simulink model "IEEE30_case"  (R2024b)
settings: Solver=FixedStepAuto  StartTime=0  StopTime=5  FixedStep=1e-7  RelTol=1e-3
values from neighbouring files (symbols this model uses):
  GFL_DFIG_7_C_bus = 0.08    [IEEE30_case_parameters.m]
  GFL_DFIG_7_D_mutual = 2.500000e+3    (= 2500)    [IEEE30_case_parameters.m]
  GFL_DFIG_7_f0 = 60    [IEEE30_case_parameters.m]
  GFL_DFIG_7_gPLLi = 3200    [IEEE30_case_parameters.m]
  GFL_DFIG_7_gPLLp = 650    [IEEE30_case_parameters.m]
  GFL_DFIG_7_H_WT = 0.4    [IEEE30_case_parameters.m]
  GFL_DFIG_7_Hg = 0.8    [IEEE30_case_parameters.m]
  GFL_DFIG_7_Igq_ref = 0    [IEEE30_case_parameters.m]
  GFL_DFIG_7_Ird_ref = 704.45696    [IEEE30_case_parameters.m]
  GFL_DFIG_7_KI_V = -300000    [IEEE30_case_parameters.m]
  GFL_DFIG_7_KP_V = -1000    [IEEE30_case_parameters.m]
  GFL_DFIG_7_Ksh = 1.254300e+4    (= 12543)    [IEEE30_case_parameters.m]
  GFL_DFIG_7_Lg = 0.000483    [IEEE30_case_parameters.m]
  GFL_DFIG_7_Lm_pu = 4    [IEEE30_case_parameters.m]
  GFL_DFIG_7_N = 100    [IEEE30_case_parameters.m]
  GFL_DFIG_7_p = 2    [IEEE30_case_parameters.m]
  GFL_DFIG_7_Pitch = 0    [IEEE30_case_parameters.m]
  GFL_DFIG_7_R = 44    [IEEE30_case_parameters.m]
  GFL_DFIG_7_Rg = 2.000000e-5    (= 2e-05)    [IEEE30_case_parameters.m]
  GFL_DFIG_7_rho = 1.225    [IEEE30_case_parameters.m]
  GFL_DFIG_7_rPLLi = 4500    [IEEE30_case_parameters.m]
  GFL_DFIG_7_rPLLp = 620    [IEEE30_case_parameters.m]
  GFL_DFIG_7_Rs_pu = 0.011    [IEEE30_case_parameters.m]
  GFL_DFIG_7_Sbase = 2.000000e+6    (= 2000000)    [IEEE30_case_parameters.m]
  GFL_DFIG_7_ugq_ref = 0    [IEEE30_case_parameters.m]
  GFL_DFIG_7_usd_ref = 0    [IEEE30_case_parameters.m]
  GFL_DFIG_7_Vbase = 690    [IEEE30_case_parameters.m]
  GFL_DFIG_7_Vdc_ref = 1200    [IEEE30_case_parameters.m]
  GFL_DFIG_7_wind = 12    [IEEE30_case_parameters.m]
  GFL_DFIG_7_wm_ref = 518.184209    [IEEE30_case_parameters.m]
  SG_D_13_D = 0.01056    [IEEE30_case_parameters.m]
  SG_D_13_EnableSaturation = 0    [IEEE30_case_parameters.m]
  SG_D_13_f0 = 60    [IEEE30_case_parameters.m]
  SG_D_13_H = 7.5    [IEEE30_case_parameters.m]
  SG_D_13_K_A = 20    [IEEE30_case_parameters.m]
  SG_D_13_K_E = 1.000000e+1    (= 10)    [IEEE30_case_parameters.m]
  SG_D_13_K_F = 2.363    [IEEE30_case_parameters.m]
  SG_D_13_K_s = 0.5    [IEEE30_case_parameters.m]
  SG_D_13_R_a = 0.001088    [IEEE30_case_parameters.m]
  SG_D_13_S_A = 1    [IEEE30_case_parameters.m]
  SG_D_13_S_B = 0.103    [IEEE30_case_parameters.m]
  SG_D_13_S_N = 10.659857    [IEEE30_case_parameters.m]
  SG_D_13_SpeedPara = 200    [IEEE30_case_parameters.m]
  SG_D_13_T_0 = 0.370163    [IEEE30_case_parameters.m]
  SG_D_13_T_1 = 0.3    [IEEE30_case_parameters.m]
  SG_D_13_T_2 = 0.05    [IEEE30_case_parameters.m]
  SG_D_13_T_3 = 0.02    [IEEE30_case_parameters.m]
  SG_D_13_T_4 = 0.005    [IEEE30_case_parameters.m]
  SG_D_13_T_A = 0.02    [IEEE30_case_parameters.m]
  SG_D_13_T_dd = 8.000000e+0    (= 8)    [IEEE30_case_parameters.m]
  SG_D_13_T_ddd = 0.04    [IEEE30_case_parameters.m]
  SG_D_13_T_E = 0.314    [IEEE30_case_parameters.m]
  SG_D_13_T_F = 0.35    [IEEE30_case_parameters.m]
  SG_D_13_T_qd = 0.8    [IEEE30_case_parameters.m]
  SG_D_13_T_qdd = 0.02    [IEEE30_case_parameters.m]
  SG_D_13_T_speed = 0.1    [IEEE30_case_parameters.m]
  SG_D_13_T_w = 0.5    [IEEE30_case_parameters.m]
  SG_D_13_V_ref = 1.696619    [IEEE30_case_parameters.m]
  SG_D_13_w_ref = 376.991118    [IEEE30_case_parameters.m]
  SG_D_13_x_d = 1.9    [IEEE30_case_parameters.m]
  SG_D_13_x_dd = 0.302    [IEEE30_case_parameters.m]
  SG_D_13_x_ddd = 0.204    [IEEE30_case_parameters.m]
  SG_D_13_x_l = 0.05    [IEEE30_case_parameters.m]
  SG_D_13_x_q = 1.3    [IEEE30_case_parameters.m]
  SG_D_13_x_qd = 0.5    [IEEE30_case_parameters.m]
  SG_D_13_x_qdd = 0.3    [IEEE30_case_parameters.m]
  SG_D_1_D = 0.01056    [IEEE30_case_parameters.m]
  SG_D_1_EnableSaturation = 0    [IEEE30_case_parameters.m]
  SG_D_1_f0 = 60    [IEEE30_case_parameters.m]
  SG_D_1_H = 7.5    [IEEE30_case_parameters.m]
  SG_D_1_K_A = 20    [IEEE30_case_parameters.m]
  SG_D_1_K_E = 1.000000e+1    (= 10)    [IEEE30_case_parameters.m]
  SG_D_1_K_F = 2.363    [IEEE30_case_parameters.m]
  SG_D_1_K_s = 0.5    [IEEE30_case_parameters.m]
  SG_D_1_R_a = 0.001088    [IEEE30_case_parameters.m]
  SG_D_1_S_A = 1    [IEEE30_case_parameters.m]
  SG_D_1_S_B = 0.103    [IEEE30_case_parameters.m]
  SG_D_1_S_N = 10.659857    [IEEE30_case_parameters.m]
  SG_D_1_SpeedPara = 200    [IEEE30_case_parameters.m]
  SG_D_1_T_0 = 0.259812    [IEEE30_case_parameters.m]
  SG_D_1_T_1 = 0.3    [IEEE30_case_parameters.m]
  SG_D_1_T_2 = 0.05    [IEEE30_case_parameters.m]
  SG_D_1_T_3 = 0.02    [IEEE30_case_parameters.m]
  SG_D_1_T_4 = 0.005    [IEEE30_case_parameters.m]
  SG_D_1_T_A = 0.02    [IEEE30_case_parameters.m]
  SG_D_1_T_dd = 8.000000e+0    (= 8)    [IEEE30_case_parameters.m]
  SG_D_1_T_ddd = 0.04    [IEEE30_case_parameters.m]
  SG_D_1_T_E = 0.314    [IEEE30_case_parameters.m]
  SG_D_1_T_F = 0.35    [IEEE30_case_parameters.m]
  SG_D_1_T_qd = 0.8    [IEEE30_case_parameters.m]
  SG_D_1_T_qdd = 0.02    [IEEE30_case_parameters.m]
  SG_D_1_T_speed = 0.1    [IEEE30_case_parameters.m]
  SG_D_1_T_w = 0.5    [IEEE30_case_parameters.m]
  SG_D_1_V_ref = 1.544107    [IEEE30_case_parameters.m]
  SG_D_1_w_ref = 376.991118    [IEEE30_case_parameters.m]
  SG_D_1_x_d = 1.9    [IEEE30_case_parameters.m]
  SG_D_1_x_dd = 0.302    [IEEE30_case_parameters.m]
  SG_D_1_x_ddd = 0.204    [IEEE30_case_parameters.m]
  SG_D_1_x_l = 0.05    [IEEE30_case_parameters.m]
  SG_D_1_x_q = 1.3    [IEEE30_case_parameters.m]
  SG_D_1_x_qd = 0.5    [IEEE30_case_parameters.m]
  SG_D_1_x_qdd = 0.3    [IEEE30_case_parameters.m]
  SG_D_22_D = 0.01056    [IEEE30_case_parameters.m]
  SG_D_22_EnableSaturation = 0    [IEEE30_case_parameters.m]
  SG_D_22_f0 = 60    [IEEE30_case_parameters.m]
  SG_D_22_H = 7.5    [IEEE30_case_parameters.m]
  SG_D_22_K_A = 20    [IEEE30_case_parameters.m]
  SG_D_22_K_E = 1.000000e+1    (= 10)    [IEEE30_case_parameters.m]
  SG_D_22_K_F = 2.363    [IEEE30_case_parameters.m]
  SG_D_22_K_s = 0.5    [IEEE30_case_parameters.m]
  SG_D_22_R_a = 0.001088    [IEEE30_case_parameters.m]
  SG_D_22_S_A = 1    [IEEE30_case_parameters.m]
  SG_D_22_S_B = 0.103    [IEEE30_case_parameters.m]
  SG_D_22_S_N = 10.659857    [IEEE30_case_parameters.m]
  SG_D_22_SpeedPara = 200    [IEEE30_case_parameters.m]
  SG_D_22_T_0 = 0.216121    [IEEE30_case_parameters.m]
  SG_D_22_T_1 = 0.3    [IEEE30_case_parameters.m]
  SG_D_22_T_2 = 0.05    [IEEE30_case_parameters.m]
  SG_D_22_T_3 = 0.02    [IEEE30_case_parameters.m]
  SG_D_22_T_4 = 0.005    [IEEE30_case_parameters.m]
  ... (+126 more)
(part 15 of 27)

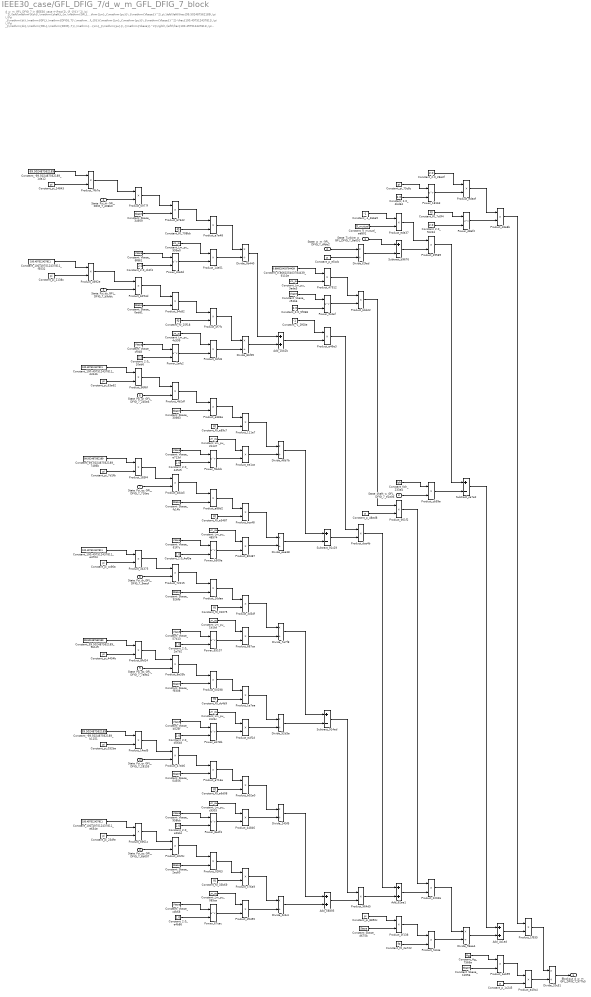
== system IEEE30_case/GFL_DFIG_7/d_w_m_GFL_DFIG_7_block ==
  note: d_w_m_GFL_DFIG_7 in IEEE30_case
      | $-\frac{2\,{f_{0}}^2\,\pi ^2\,\left(\mathrm{Ksh}\,\mathrm{shaft}_{w,\mathrm{GFL},\mathrm{DFIG},7}+D_{\mathrm{mutual}}\,\left(\mathrm{Turbine}_{w,\mathrm{GFL},\mathrm{DFIG},7}-\frac{w_{m,\mathrm{GFL},\mathrm{DFIG},7}}{p}\right)-\frac{0.866025403784439\,\mathrm{Lm}_{\mathrm{pu}}\,{\mathrm{Vbase}}^2\,p\,\left(\left(\frac{99.502487562189\,\pi \,\Psi _{\mathrm{dr},\mathrm{GFL},\mathrm{DFIG},7}\,\mathrm{Sbase}\,f_{0}}{\mathrm{Lm}_{\mathrm{pu}}\,{\mathrm{Vbase}}^2}-\frac{100.497512437811\,\pi \,\Psi _{\mathrm{ds},\mathrm{GFL},\mathrm{DFIG},7}\,\mathrm{Sbase}\,f_{0}}{\mathrm{Lm}_{\mathrm{pu}}\,{\mathrm{Vbase}}^2}\right)\,\left(\frac{100.497512437811\,\pi \,\Psi _{\mathrm{qr},\mathrm{GFL},\mathrm{DFIG},7}\,\mathrm{Sbase}\,f_{0}}{\mathrm{Lm}_{\mathrm{pu}}\,{\mathrm{Vbase}}^2}-\frac{99.502487562189\,\pi \,\Psi _{\mathrm{qs},\mathrm{GFL},\mathrm{DFIG},7}\,\mathrm{Sbase}\,f_{0}}{\mathrm{Lm}_{\mathrm{pu}}\,{\mathrm{Vbase}}^2}\right)-\left(\frac{100.497512437811\,\pi \,\Psi _{\mathrm{dr},\mathrm{GFL},\mathrm{DFIG},7}\,\mathrm{Sbase}\,f_{0}}{\mathrm{Lm}_{\mathrm{pu}}\,{\mathrm{Vbase}}^2}-\frac{99.502487562189\,\pi \,\Psi _{\mathrm{ds},\mathrm{GFL},\mathrm{DFIG},7}\,\mathrm{Sbase}\,f_{0}}{\mathrm{Lm}_{\mathrm{pu}}\,{\mathrm{Vbase}}^2}\right)\,\left(\frac{99.502487562189\,\pi \,\Psi _{\mathrm{qr},\mathrm{GFL},\mathrm{DFIG},7}\,\mathrm{Sbase}\,f_{0}}{\mathrm{Lm}_{\mathrm{pu}}\,{\mathrm{Vbase}}^2}-\frac{100.497512437811\,\pi \,\Psi _{\mathrm{qs},\mathrm{GFL},\mathrm{DFIG},7}\,\mathrm{Sbase}\,f_{0}}{\mathrm{Lm}_{\mathrm{pu}}\,{\mathrm{Vbase}}^2}\right)\right)}{\mathrm{Sbase}\,f_{0}\,\pi }\right)}{\mathrm{Hg}\,\mathrm{Sbase}\,p}$
      | Automatically generated on 2025-11-01 18:32:24 .
  State_Turbine_w_GFL_DFIG_7_8e651 : Inport
  State_w_m_GFL_DFIG_7_dfde2 : Inport  Port=2
  State_shaft_w_GFL_DFIG_7_e1a06 : Inport  Port=3
  State_Psi_dr_GFL_DFIG_7_d08b0 : Inport  Port=4
  State_Psi_ds_GFL_DFIG_7_b9ddc : Inport  Port=5
  State_Psi_qr_GFL_DFIG_7_240a6 : Inport  Port=6
  State_Psi_qs_GFL_DFIG_7_716ac : Inport  Port=7
  State_Psi_dr_GFL_DFIG_7_9aecf : Inport  Port=8
  State_Psi_ds_GFL_DFIG_7_7aea2 : Inport  Port=9
  State_Psi_qr_GFL_DFIG_7_28155 : Inport  Port=10
  State_Psi_qs_GFL_DFIG_7_6b007 : Inport  Port=11
  Add_1bb2b : Sum
  Add_4c1ed : Sum
  Add_58d95 : Sum
  Add_62ae1 : Sum
  Constant_-1_2f60e : Constant  Value=-1
  Constant_-1_466a5 : Constant  Value=-1
  Constant_-99.502487562189_1da12 : Constant  Value=-99.502487562189
  Constant_-99.502487562189_b1151 : Constant  Value=-99.502487562189
  Constant_0.866025403784439_9110e : Constant  Value=0.866025403784439
  Constant_100.497512437811_dd14b : Constant  Value=100.497512437811
  Constant_100.497512437811_e4704 : Constant  Value=100.497512437811
  Constant_100.497512437811_e654e : Constant  Value=100.497512437811
  Constant_100.497512437811_f5532 : Constant  Value=100.497512437811
  Constant_2.0_10ab6 : Constant  Value=2.0
  Constant_2.0_28e3f : Constant  Value=2.0
  Constant_2.0_2a7b2 : Constant  Value=2.0
  Constant_2.0_445c5 : Constant  Value=2.0
  Constant_2.0_4bd64 : Constant  Value=2.0
  Constant_2.0_4ef5a : Constant  Value=2.0
  Constant_2.0_5f068 : Constant  Value=2.0
  Constant_2.0_9c243 : Constant  Value=2.0
  Constant_2.0_cb1f4 : Constant  Value=2.0
  Constant_2.0_d56bd : Constant  Value=2.0
  Constant_2.0_e26bc : Constant  Value=2.0
  Constant_2.0_e4b86 : Constant  Value=2.0
  Constant_99.502487562189_7486b : Constant  Value=99.502487562189
  Constant_99.502487562189_9b1c9 : Constant  Value=99.502487562189
  Constant_D_mutual_aed01 : Constant  Value=D_mutual
  Constant_Hg_7566a : Constant  Value=Hg
  Constant_Ksh_233a4 : Constant  Value=Ksh
  Constant_Lm_pu_085ca : Constant  Value=Lm_pu
  Constant_Lm_pu_1b1cd : Constant  Value=Lm_pu
  Constant_Lm_pu_2b137 : Constant  Value=Lm_pu
  Constant_Lm_pu_2c24c : Constant  Value=Lm_pu
  Constant_Lm_pu_3ade3 : Constant  Value=Lm_pu
  Constant_Lm_pu_48574 : Constant  Value=Lm_pu
  Constant_Lm_pu_4c599 : Constant  Value=Lm_pu
  Constant_Lm_pu_999a0 : Constant  Value=Lm_pu
  Constant_Lm_pu_c9303 : Constant  Value=Lm_pu
  Constant_Sbase_04556 : Constant  Value=Sbase
  Constant_Sbase_0add1 : Constant  Value=Sbase
  Constant_Sbase_1b556 : Constant  Value=Sbase
  Constant_Sbase_2ec60 : Constant  Value=Sbase
  Constant_Sbase_30983 : Constant  Value=Sbase
  Constant_Sbase_34959 : Constant  Value=Sbase
  Constant_Sbase_926fb : Constant  Value=Sbase
  Constant_Sbase_d675b : Constant  Value=Sbase
  Constant_Sbase_f9308 : Constant  Value=Sbase
  Constant_Sbase_fc14b : Constant  Value=Sbase
  Constant_Vbase_57b13 : Constant  Value=Vbase
  Constant_Vbase_61f7c : Constant  Value=Vbase
  Constant_Vbase_6f861 : Constant  Value=Vbase
  Constant_Vbase_958bb : Constant  Value=Vbase
  Constant_Vbase_b526f : Constant  Value=Vbase
  Constant_Vbase_c53b6 : Constant  Value=Vbase
  Constant_Vbase_cdb68 : Constant  Value=Vbase
  Constant_Vbase_cf948 : Constant  Value=Vbase
  Constant_Vbase_e713d : Constant  Value=Vbase
  Constant_f0_01075 : Constant  Value=f0
  Constant_f0_25f18 : Constant  Value=f0
  Constant_f0_2e722 : Constant  Value=f0
  Constant_f0_33b69 : Constant  Value=f0
  Constant_f0_708bb : Constant  Value=f0
  Constant_f0_7c0f4 : Constant  Value=f0
  Constant_f0_a3487 : Constant  Value=f0
  Constant_f0_a6d08 : Constant  Value=f0
  Constant_f0_dc4b9 : Constant  Value=f0
  Constant_f0_e89c7 : Constant  Value=f0
  Constant_p_1c245 : Constant  Value=p
  Constant_p_48ad8 : Constant  Value=p
  Constant_p_e5cdc : Constant  Value=p
  Constant_pi_032ba : Constant  Value=pi
  Constant_pi_2138c : Constant  Value=pi
  Constant_pi_23dfe : Constant  Value=pi
  Constant_pi_24843 : Constant  Value=pi
  Constant_pi_4454b : Constant  Value=pi
  Constant_pi_63a62 : Constant  Value=pi
  Constant_pi_75c8c : Constant  Value=pi
  Constant_pi_7d1fb : Constant  Value=pi
  Constant_pi_8850c : Constant  Value=pi
  Constant_pi_cc96a : Constant  Value=pi
  Divide_0b440 : Product  Inputs=*/
  Divide_0c4cc : Product  Inputs=*/
  Divide_20c51 : Product  Inputs=*/
  Divide_245f5 : Product  Inputs=*/
  Divide_46b7b : Product  Inputs=*/
  Divide_52d3a : Product  Inputs=*/
  Divide_7e7f8 : Product  Inputs=*/
  Divide_8bf05 : Product  Inputs=*/
  Divide_96aa4 : Product  Inputs=*/
  Divide_eaa38 : Product  Inputs=*/
  Divide_f2fed : Product  Inputs=*/
  Power_18163 : Math  Operator=pow
  Power_2afc2 : Math  Operator=pow
  Power_3ca0d : Math  Operator=pow
  Power_65107 : Math  Operator=pow
  Power_67cac : Math  Operator=pow
  Power_8adf3 : Math  Operator=pow
  Power_9bdcb : Math  Operator=pow
  Power_9c4ef : Math  Operator=pow
  Power_b500e : Math  Operator=pow
  Power_d8ef2 : Math  Operator=pow
  Power_eb78b : Math  Operator=pow
  Product_00298 : Product
  Product_02f63 : Product
  Product_0977f : Product
  Product_0cfc8 : Product
  Product_111e7 : Product
  Product_14ad5 : Product
  Product_14e51 : Product
  Product_16daa : Product
  Product_183f4 : Product
  Product_1e7aa : Product
  Product_1eb99 : Product
  Product_1f935 : Product
  Product_{22046,34375,44846,47912,49589,67642,72215,80487} (8 alike) : Product
  Product_3d3df : Product
  Product_3f138 : Product
  Product_47ab6 : Product
  Product_484c5 : Product
  Product_4992e : Product
  Product_4b2df : Product
  Product_4f7fc : Product
  Product_6294d : Product
  Product_7fb7e : Product
  Product_887ca : Product
  Product_8a33b : Product
  Product_8fd24 : Product
  Product_901f2 : Product
  Product_94c82 : Product
  Product_964d5 : Product
  Product_96f6f : Product
  Product_a49c4 : Product
  Product_a4f1d : Product
  Product_a716a : Product
  Product_a88d2 : Product
  Product_b02a0 : Product
  Product_b961c : Product
  Product_bbb22 : Product
  Product_bcc48 : Product
  Product_c76a9 : Product
  Product_cb99a : Product
  Product_d2c5c : Product
  Product_d3a8b : Product
  Product_d5455 : Product
  Product_dce4b : Product
  Product_e383e : Product
  Product_e46e3 : Product
  Product_e7a48 : Product
  Product_eda37 : Product
  Product_edaaf : Product
  Product_ee1ca : Product
  Product_f4c4e : Product
  Subtract_914ed : Sum  Inputs=+-
  Subtract_91c29 : Sum  Inputs=+-
  Subtract_b9676 : Sum  Inputs=+-
  Subtract_ca7e2 : Sum  Inputs=+-
  Blockout_d_w_m_GFL_DFIG_7_977b5 : Outport
  wires:
  Product_1eb99/1 -> Product_a49c4/1
  Add_4c1ed/1 -> Product_1f935/2
  Divide_20c51/1 -> Blockout_d_w_m_GFL_DFIG_7_977b5/1
  Product_16daa/1 -> Product_3d3df/1
  Constant_2.0_4ef5a/1 -> Power_b500e/2
  Constant_-99.502487562189_b1151/1 -> Product_14ad5/1
  Add_62ae1/1 -> Product_22046/2
  Product_a49c4/1 -> Divide_20c51/2
  Constant_Vbase_b526f/1 -> Power_eb78b/1
  Constant_-1_2f60e/1 -> Product_e46e3/1
  Product_44846/1 -> Divide_245f5/2
  Product_22046/1 -> Divide_96aa4/1
  Product_1f935/1 -> Divide_20c51/1
  Constant_p_1c245/1 -> Product_a49c4/2
  Constant_99.502487562189_9b1c9/1 -> Product_8fd24/1
  Add_58d95/1 -> Product_964d5/2
  Product_964d5/1 -> Add_62ae1/2
  Product_f4c4e/1 -> Divide_96aa4/2
  Product_d5455/1 -> Divide_0c4cc/2
  Subtract_91c29/1 -> Product_dce4b/2
  Constant_2.0_4bd64/1 -> Power_18163/2
  Constant_Sbase_1b556/1 -> Product_1eb99/2
  Divide_eaa38/1 -> Subtract_91c29/2
  Constant_Hg_7566a/1 -> Product_1eb99/1
  Constant_Sbase_2ec60/1 -> Product_02f63/2
  Constant_Vbase_958bb/1 -> Power_8adf3/1
  Divide_0c4cc/1 -> Add_58d95/2
  Constant_2.0_28e3f/1 -> Product_edaaf/1
  Product_a4f1d/1 -> Divide_52d3a/2
  Constant_Lm_pu_48574/1 -> Product_80487/1
  Constant_Sbase_30983/1 -> Product_e383e/2
  Product_b961c/1 -> Product_d2c5c/1
  State_shaft_w_GFL_DFIG_7_e1a06/1 -> Product_cb99a/2
  Divide_96aa4/1 -> Add_4c1ed/2
  Constant_Lm_pu_2c24c/1 -> Product_a4f1d/1
  Constant_Sbase_926fb/1 -> Product_16daa/2
  Product_d2c5c/1 -> Product_02f63/1
  Product_c76a9/1 -> Divide_0c4cc/1
  Power_9c4ef/1 -> Product_bbb22/2
  Constant_pi_8850c/1 -> Product_3f138/1
  Constant_f0_2e722/1 -> Product_f4c4e/2
  Constant_f0_e89c7/1 -> Product_111e7/2
  Product_3f138/1 -> Product_f4c4e/1
  Product_4b2df/1 -> Product_e383e/1
  Constant_2.0_e26bc/1 -> Power_8adf3/2
  State_Psi_dr_GFL_DFIG_7_d08b0/1 -> Product_0977f/2
  Constant_Sbase_d675b/1 -> Product_3f138/2
  Product_8a33b/1 -> Product_00298/1
  Constant_pi_032ba/1 -> Product_14ad5/2
  Constant_Vbase_cdb68/1 -> Power_67cac/1
  Divide_245f5/1 -> Add_58d95/1
  Constant_Lm_pu_c9303/1 -> Product_44846/1
  Product_3d3df/1 -> Divide_7e7f8/1
  Power_67cac/1 -> Product_d5455/2
  State_Psi_ds_GFL_DFIG_7_7aea2/1 -> Product_8a33b/2
  Product_96f6f/1 -> Product_4b2df/1
  Constant_2.0_e4b86/1 -> Power_67cac/2
  Divide_8bf05/1 -> Add_1bb2b/2
  Constant_Lm_pu_085ca/1 -> Product_d5455/1
  Constant_pi_2138c/1 -> Product_4992e/2
  Constant_f0_33b69/1 -> Product_c76a9/2
  Product_02f63/1 -> Product_c76a9/1
  Power_8adf3/1 -> Product_44846/2
  State_Psi_qs_GFL_DFIG_7_6b007/1 -> Product_d2c5c/2
  Constant_100.497512437811_e654e/1 -> Product_b961c/1
  Constant_Sbase_f9308/1 -> Product_00298/2
  Constant_pi_23dfe/1 -> Product_b961c/2
  Product_8fd24/1 -> Product_8a33b/1
  State_Psi_qr_GFL_DFIG_7_28155/1 -> Product_47ab6/2
  State_Psi_qs_GFL_DFIG_7_716ac/1 -> Product_484c5/2
  State_Turbine_w_GFL_DFIG_7_8e651/1 -> Subtract_b9676/1
  Constant_Sbase_fc14b/1 -> Product_a88d2/2
  Product_b02a0/1 -> Divide_245f5/1
  Power_eb78b/1 -> Product_a4f1d/2
  Subtract_914ed/1 -> Product_964d5/1
  Constant_f0_a6d08/1 -> Product_b02a0/2
  Product_a716a/1 -> Product_b02a0/1
  Constant_2.0_5f068/1 -> Power_9c4ef/2
  Constant_Sbase_04556/1 -> Product_a716a/2
  Constant_f0_dc4b9/1 -> Product_1e7aa/2
  Product_47ab6/1 -> Product_a716a/1
  Product_eda37/1 -> Product_49589/1
  Product_80487/1 -> Divide_eaa38/2
  Product_14ad5/1 -> Product_47ab6/1
  Product_00298/1 -> Product_1e7aa/1
  Divide_52d3a/1 -> Subtract_914ed/2
  Constant_2.0_d56bd/1 -> Power_eb78b/2
  Product_1e7aa/1 -> Divide_52d3a/1
  Constant_pi_4454b/1 -> Product_8fd24/2
  Divide_7e7f8/1 -> Subtract_914ed/1
  Product_887ca/1 -> Divide_7e7f8/2
  Power_65107/1 -> Product_887ca/2
  Constant_pi_75c8c/1 -> Power_18163/1
  Constant_2.0_2a7b2/1 -> Power_65107/2
  Constant_Vbase_57b13/1 -> Power_65107/1
  Constant_Lm_pu_1b1cd/1 -> Product_887ca/1
  Constant_f0_01075/1 -> Product_3d3df/2
  Product_72215/1 -> Product_16daa/1
  State_Psi_dr_GFL_DFIG_7_9aecf/1 -> Product_72215/2
  Product_34375/1 -> Product_72215/1
  Constant_pi_cc96a/1 -> Product_34375/2
  Constant_100.497512437811_e4704/1 -> Product_34375/1
  Product_d3a8b/1 -> Product_1f935/1
  Product_dce4b/1 -> Add_62ae1/1
  Power_b500e/1 -> Product_80487/2
  Constant_Vbase_61f7c/1 -> Power_b500e/1
  Product_bcc48/1 -> Divide_eaa38/1
  Constant_f0_a3487/1 -> Product_bcc48/2
  Product_a88d2/1 -> Product_bcc48/1
  Subtract_ca7e2/1 -> Add_4c1ed/1
  Product_484c5/1 -> Product_a88d2/1
  Product_183f4/1 -> Product_484c5/1
  Constant_2.0_9c243/1 -> Power_d8ef2/2
  Constant_pi_7d1fb/1 -> Product_183f4/2
  Constant_99.502487562189_7486b/1 -> Product_183f4/1
  Divide_46b7b/1 -> Subtract_91c29/1
  Divide_f2fed/1 -> Subtract_b9676/2
  Product_ee1ca/1 -> Divide_46b7b/2
  Power_9bdcb/1 -> Product_ee1ca/2
  Constant_2.0_445c5/1 -> Power_9bdcb/2
  Constant_Vbase_e713d/1 -> Power_9bdcb/1
  State_w_m_GFL_DFIG_7_dfde2/1 -> Divide_f2fed/1
  Constant_Lm_pu_2b137/1 -> Product_ee1ca/1
  Product_111e7/1 -> Divide_46b7b/1
  Product_e383e/1 -> Product_111e7/1
  State_Psi_qr_GFL_DFIG_7_240a6/1 -> Product_4b2df/2
  Constant_pi_63a62/1 -> Product_96f6f/2
  Constant_100.497512437811_dd14b/1 -> Product_96f6f/1
  Product_e46e3/1 -> Product_dce4b/1
  Add_1bb2b/1 -> Product_e46e3/2
  Product_0cfc8/1 -> Divide_8bf05/2
  Power_2afc2/1 -> Product_0cfc8/2
  Constant_2.0_10ab6/1 -> Power_2afc2/2
  Constant_Vbase_cf948/1 -> Power_2afc2/1
  Constant_Sbase_34959/1 -> Product_67642/2
  Constant_Lm_pu_4c599/1 -> Product_0cfc8/1
  Product_e7a48/1 -> Divide_0b440/1
  Product_4f7fc/1 -> Divide_8bf05/1
  Constant_f0_25f18/1 -> Product_4f7fc/2
  Product_94c82/1 -> Product_4f7fc/1
  Constant_Sbase_0add1/1 -> Product_94c82/2
  Product_6294d/1 -> Product_94c82/1
  State_Psi_ds_GFL_DFIG_7_b9ddc/1 -> Product_6294d/2
  Product_4992e/1 -> Product_6294d/1
  Constant_100.497512437811_f5532/1 -> Product_4992e/1
  Divide_0b440/1 -> Add_1bb2b/1
  Product_14e51/1 -> Divide_0b440/2
  Power_3ca0d/1 -> Product_14e51/2
  Constant_2.0_cb1f4/1 -> Power_3ca0d/2
  Constant_Vbase_6f861/1 -> Power_3ca0d/1
  Constant_Lm_pu_999a0/1 -> Product_14e51/1
  Constant_f0_708bb/1 -> Product_e7a48/2
  Product_67642/1 -> Product_e7a48/1
  Constant_p_e5cdc/1 -> Divide_f2fed/2
  Product_0977f/1 -> Product_67642/1
  Product_7fb7e/1 -> Product_0977f/1
  Constant_pi_24843/1 -> Product_7fb7e/2
  Constant_-99.502487562189_1da12/1 -> Product_7fb7e/1
  Product_901f2/1 -> Product_22046/1
  Constant_p_48ad8/1 -> Product_901f2/2
  Product_bbb22/1 -> Product_901f2/1
  Constant_Vbase_c53b6/1 -> Power_9c4ef/1
  Product_47912/1 -> Product_bbb22/1
  Constant_Lm_pu_3ade3/1 -> Product_47912/2
  Constant_0.866025403784439_9110e/1 -> Product_47912/1
  Product_cb99a/1 -> Subtract_ca7e2/2
  Constant_Ksh_233a4/1 -> Product_cb99a/1
  Product_49589/1 -> Subtract_ca7e2/1
  Subtract_b9676/1 -> Product_49589/2
  Constant_D_mutual_aed01/1 -> Product_eda37/2
  Constant_-1_466a5/1 -> Product_eda37/1
  Power_d8ef2/1 -> Product_d3a8b/2
  Constant_f0_7c0f4/1 -> Power_d8ef2/1
  Product_edaaf/1 -> Product_d3a8b/1
  Power_18163/1 -> Product_edaaf/2

== system IEEE30_case/GFL_DFIG_7/i_d_GFL_DFIG_7_block ==
  note: i_d_GFL_DFIG_7 in IEEE30_case
      | $-\frac{0.0000345\,\mathrm{Sbase}\,\left(\frac{1.73205080756888\,\mathrm{Vbase}\,\left(\cos\left(\theta _{\mathrm{pllr},\mathrm{GFL},\mathrm{DFIG},7}\right)\,\left(\frac{99.502487562189\,\pi \,\Psi _{\mathrm{dr},\mathrm{GFL},\mathrm{DFIG},7}\,\mathrm{Sbase}\,f_{0}}{\mathrm{Lm}_{\mathrm{pu}}\,{\mathrm{Vbase}}^2}-\frac{100.497512437811\,\pi \,\Psi _{\mathrm{ds},\mathrm{GFL},\mathrm{DFIG},7}\,\mathrm{Sbase}\,f_{0}}{\mathrm{Lm}_{\mathrm{pu}}\,{\mathrm{Vbase}}^2}\right)+\sin\left(\theta _{\mathrm{pllr},\mathrm{GFL},\mathrm{DFIG},7}\right)\,\left(\frac{99.502487562189\,\pi \,\Psi _{\mathrm{qr},\mathrm{GFL},\mathrm{DFIG},7}\,\mathrm{Sbase}\,f_{0}}{\mathrm{Lm}_{\mathrm{pu}}\,{\mathrm{Vbase}}^2}-\frac{100.497512437811\,\pi \,\Psi _{\mathrm{qs},\mathrm{GFL},\mathrm{DFIG},7}\,\mathrm{Sbase}\,f_{0}}{\mathrm{Lm}_{\mathrm{pu}}\,{\mathrm{Vbase}}^2}\right)\right)}{\mathrm{Sbase}}-\frac{1.73205080756888\,\mathrm{Vbase}\,\left(i_{\mathrm{gd},\mathrm{GFL},\mathrm{DFIG},7}\,\cos\left(\theta _{\mathrm{pllg},\mathrm{GFL},\mathrm{DFIG},7}\right)+i_{\mathrm{gq},\mathrm{GFL},\mathrm{DFIG},7}\,\sin\left(\theta _{\mathrm{pllg},\mathrm{GFL},\mathrm{DFIG},7}\right)\right)}{\mathrm{Sbase}}\right)}{\mathrm{Vbase}}$
      | Automatically generated on 2025-11-01 18:34:14 .
  State_i_gd_GFL_DFIG_7_c7c38 : Inport
  State_theta_pllg_GFL_DFIG_7_3c4e6 : Inport  Port=2
  State_i_gq_GFL_DFIG_7_12231 : Inport  Port=3
  State_theta_pllg_GFL_DFIG_7_99cce : Inport  Port=4
  State_Psi_dr_GFL_DFIG_7_47f96 : Inport  Port=5
  State_Psi_ds_GFL_DFIG_7_8722f : Inport  Port=6
  State_theta_pllr_GFL_DFIG_7_79db7 : Inport  Port=7
  State_Psi_qr_GFL_DFIG_7_2c5a7 : Inport  Port=8
  State_Psi_qs_GFL_DFIG_7_a1324 : Inport  Port=9
  State_theta_pllr_GFL_DFIG_7_e04ad : Inport  Port=10
  Add_492a2 : Sum
  Add_49bd1 : Sum
  Add_e7d18 : Sum
  Constant_-1_c11df : Constant  Value=-1
  Constant_-5.0_f5269 : Constant  Value=-5.0
  Constant_-99.502487562189_65d39 : Constant  Value=-99.502487562189
  Constant_-99.502487562189_e1ca6 : Constant  Value=-99.502487562189
  Constant_1.73205080756888_ce066 : Constant  Value=1.73205080756888
  Constant_1.73205080756888_e9173 : Constant  Value=1.73205080756888
  Constant_10.0_49afa : Constant  Value=10.0
  Constant_100.497512437811_8d135 : Constant  Value=100.497512437811
  Constant_100.497512437811_9df18 : Constant  Value=100.497512437811
  Constant_2.0_2fdd8 : Constant  Value=2.0
  Constant_2.0_40610 : Constant  Value=2.0
  Constant_2.0_40c81 : Constant  Value=2.0
  Constant_2.0_c02d0 : Constant  Value=2.0
  Constant_3.45_a6674 : Constant  Value=3.45
  Constant_Lm_pu_2dd3f : Constant  Value=Lm_pu
  Constant_Lm_pu_78702 : Constant  Value=Lm_pu
  Constant_Lm_pu_cb21c : Constant  Value=Lm_pu
  Constant_Lm_pu_edadb : Constant  Value=Lm_pu
  Constant_Sbase_0edc5 : Constant  Value=Sbase
  Constant_Sbase_30f20 : Constant  Value=Sbase
  Constant_Sbase_5a1d3 : Constant  Value=Sbase
  Constant_Sbase_9d97b : Constant  Value=Sbase
  Constant_Sbase_d8b83 : Constant  Value=Sbase
  Constant_Sbase_de693 : Constant  Value=Sbase
  Constant_Sbase_fbf63 : Constant  Value=Sbase
  Constant_Vbase_00e0b : Constant  Value=Vbase
  Constant_Vbase_4dc36 : Constant  Value=Vbase
  Constant_Vbase_65299 : Constant  Value=Vbase
  Constant_Vbase_67351 : Constant  Value=Vbase
  Constant_Vbase_97988 : Constant  Value=Vbase
  Constant_Vbase_f62ff : Constant  Value=Vbase
  Constant_Vbase_fa0fe : Constant  Value=Vbase
  Constant_f0_58a72 : Constant  Value=f0
  Constant_f0_75a91 : Constant  Value=f0
  Constant_f0_844bc : Constant  Value=f0
  Constant_f0_94819 : Constant  Value=f0
  Constant_pi_0046d : Constant  Value=pi
  Constant_pi_07071 : Constant  Value=pi
  Constant_pi_98dd5 : Constant  Value=pi
  Constant_pi_ee553 : Constant  Value=pi
  Divide_1a3a0 : Product  Inputs=*/
  Divide_7078c : Product  Inputs=*/
  Divide_7cc1f : Product  Inputs=*/
  Divide_9a0f6 : Product  Inputs=*/
  Divide_c73cd : Product  Inputs=*/
  Divide_d7e58 : Product  Inputs=*/
  Divide_ed1b1 : Product  Inputs=*/
  MathFunc_cos_b7057 : Trigonometry  Operator=cos
  MathFunc_cos_c2863 : Trigonometry  Operator=cos
  MathFunc_sin_bdbfa : Trigonometry
  MathFunc_sin_fb6a3 : Trigonometry
  Power_4816e : Math  Operator=pow
  Power_82469 : Math  Operator=pow
  Power_8f089 : Math  Operator=pow
  Power_98ba8 : Math  Operator=pow
  Power_9e004 : Math  Operator=pow
  Product_07985 : Product
  Product_0fc16 : Product
  Product_1b707 : Product
  Product_24ce9 : Product
  Product_2c6cc : Product
  Product_31851 : Product
  Product_38eb7 : Product
  Product_3fff3 : Product
  Product_4f502 : Product
  Product_5ad5c : Product
  Product_5c8fa : Product
  Product_653a1 : Product
  Product_6c949 : Product
  Product_71635 : Product
  Product_7859f : Product
  Product_7fea7 : Product
  Product_925c3 : Product
  Product_a23e8 : Product
  Product_a2ec9 : Product
  Product_a485c : Product
  Product_aeb12 : Product
  Product_b0865 : Product
  Product_b1903 : Product
  Product_b70ed : Product
  Product_beed1 : Product
  Product_c30f9 : Product
  Product_db37c : Product
  Product_de865 : Product
  Product_dfd1d : Product
  Product_e0cff : Product
  Product_e5dbc : Product
  Product_fe51d : Product
  Subtract_62b79 : Sum  Inputs=+-
  Subtract_a4cea : Sum  Inputs=+-
  Blockout_i_d_GFL_DFIG_7_2a8ae : Outport
  wires:
  Constant_-99.502487562189_e1ca6/1 -> Product_7859f/1
  State_Psi_dr_GFL_DFIG_7_47f96/1 -> Product_5ad5c/2
  Constant_100.497512437811_9df18/1 -> Product_fe51d/1
  State_Psi_ds_GFL_DFIG_7_8722f/1 -> Product_db37c/2
  Constant_pi_ee553/1 -> Product_7859f/2
  Constant_100.497512437811_8d135/1 -> Product_653a1/1
  Divide_d7e58/1 -> Subtract_62b79/2
  Constant_pi_0046d/1 -> Product_fe51d/2
  Product_5c8fa/1 -> Divide_c73cd/1
  Product_7859f/1 -> Product_5ad5c/1
  State_theta_pllg_GFL_DFIG_7_99cce/1 -> MathFunc_sin_bdbfa/1
  Product_b0865/1 -> Divide_9a0f6/1
  Product_fe51d/1 -> Product_db37c/1
  Constant_-99.502487562189_65d39/1 -> Product_aeb12/1
  Constant_2.0_40c81/1 -> Power_98ba8/2
  Product_71635/1 -> Product_4f502/1
  Constant_pi_98dd5/1 -> Product_aeb12/2
  Product_b70ed/1 -> Product_31851/1
  Constant_pi_07071/1 -> Product_653a1/2
  Divide_c73cd/1 -> Add_e7d18/1
  State_Psi_qr_GFL_DFIG_7_2c5a7/1 -> Product_e0cff/2
  Product_5ad5c/1 -> Product_71635/1
  Constant_Sbase_30f20/1 -> Product_71635/2
  Constant_Vbase_67351/1 -> Power_4816e/1
  Product_0fc16/1 -> Divide_c73cd/2
  Constant_2.0_c02d0/1 -> Power_4816e/2
  State_Psi_qs_GFL_DFIG_7_a1324/1 -> Product_b70ed/2
  Product_db37c/1 -> Product_a23e8/1
  Constant_Sbase_0edc5/1 -> Product_a23e8/2
  Constant_Vbase_65299/1 -> Power_82469/1
  Constant_f0_94819/1 -> Product_b0865/2
  Constant_2.0_40610/1 -> Power_82469/2
  Product_aeb12/1 -> Product_e0cff/1
  Product_653a1/1 -> Product_b70ed/1
  Constant_10.0_49afa/1 -> Power_9e004/1
  Constant_f0_844bc/1 -> Product_4f502/2
  Constant_Lm_pu_78702/1 -> Product_dfd1d/1
  Power_4816e/1 -> Product_dfd1d/2
  Constant_Sbase_d8b83/1 -> Product_31851/2
  Product_a23e8/1 -> Product_e5dbc/1
  State_i_gq_GFL_DFIG_7_12231/1 -> Product_3fff3/1
  Constant_f0_58a72/1 -> Product_e5dbc/2
  Constant_Lm_pu_cb21c/1 -> Product_24ce9/1
  Power_82469/1 -> Product_24ce9/2
  Product_e0cff/1 -> Product_a2ec9/1
  Constant_Sbase_5a1d3/1 -> Product_a2ec9/2
  State_theta_pllg_GFL_DFIG_7_3c4e6/1 -> MathFunc_cos_b7057/1
  Divide_ed1b1/1 -> Add_492a2/2
  Constant_Vbase_00e0b/1 -> Power_8f089/1
  Constant_2.0_2fdd8/1 -> Power_8f089/2
  Power_8f089/1 -> Product_0fc16/2
  Constant_Vbase_97988/1 -> Power_98ba8/1
  Product_4f502/1 -> Divide_1a3a0/1
  Product_dfd1d/1 -> Divide_1a3a0/2
  Product_e5dbc/1 -> Divide_ed1b1/1
  Product_24ce9/1 -> Divide_ed1b1/2
  Product_a2ec9/1 -> Product_5c8fa/1
  Power_98ba8/1 -> Product_925c3/2
  Constant_Lm_pu_2dd3f/1 -> Product_0fc16/1
  Constant_f0_75a91/1 -> Product_5c8fa/2
  Product_31851/1 -> Product_b0865/1
  Constant_Lm_pu_edadb/1 -> Product_925c3/1
  Divide_1a3a0/1 -> Add_492a2/1
  Product_1b707/1 -> Product_7fea7/1
  Product_925c3/1 -> Divide_9a0f6/2
  Constant_-1_c11df/1 -> Product_beed1/1
  State_theta_pllr_GFL_DFIG_7_79db7/1 -> MathFunc_cos_c2863/1
  Add_492a2/1 -> Product_beed1/2
  Divide_9a0f6/1 -> Add_e7d18/2
  State_theta_pllr_GFL_DFIG_7_e04ad/1 -> MathFunc_sin_fb6a3/1
  State_i_gd_GFL_DFIG_7_c7c38/1 -> Product_a485c/1
  MathFunc_cos_b7057/1 -> Product_a485c/2
  MathFunc_sin_bdbfa/1 -> Product_3fff3/2
  Product_beed1/1 -> Product_b1903/1
  MathFunc_cos_c2863/1 -> Product_b1903/2
  Add_e7d18/1 -> Product_07985/1
  MathFunc_sin_fb6a3/1 -> Product_07985/2
  Constant_1.73205080756888_e9173/1 -> Product_38eb7/1
  Constant_Vbase_f62ff/1 -> Product_38eb7/2
  Product_a485c/1 -> Add_49bd1/1
  Product_3fff3/1 -> Add_49bd1/2
  Constant_1.73205080756888_ce066/1 -> Product_1b707/1
  Constant_Vbase_fa0fe/1 -> Product_1b707/2
  Product_b1903/1 -> Subtract_a4cea/1
  Product_07985/1 -> Subtract_a4cea/2
  Constant_-5.0_f5269/1 -> Power_9e004/2
  Product_38eb7/1 -> Product_2c6cc/1
  Product_de865/1 -> Divide_7078c/1
  Add_49bd1/1 -> Product_2c6cc/2
  Subtract_a4cea/1 -> Product_7fea7/2
  Constant_3.45_a6674/1 -> Product_6c949/1
  Power_9e004/1 -> Product_6c949/2
  Product_2c6cc/1 -> Divide_7cc1f/1
  Constant_Sbase_de693/1 -> Divide_7cc1f/2
  Product_7fea7/1 -> Divide_d7e58/1
  Constant_Sbase_fbf63/1 -> Divide_d7e58/2
  Product_6c949/1 -> Product_c30f9/1
  Constant_Sbase_9d97b/1 -> Product_c30f9/2
  Divide_7078c/1 -> Blockout_i_d_GFL_DFIG_7_2a8ae/1
  Divide_7cc1f/1 -> Subtract_62b79/1
  Product_c30f9/1 -> Product_de865/1
  Subtract_62b79/1 -> Product_de865/2
  Constant_Vbase_4dc36/1 -> Divide_7078c/2

== system IEEE30_case/GFL_DFIG_7/i_q_GFL_DFIG_7_block ==
  note: i_q_GFL_DFIG_7 in IEEE30_case
      | $-\frac{0.0000345\,\mathrm{Sbase}\,\left(\frac{1.73205080756888\,\mathrm{Vbase}\,\left(\cos\left(\theta _{\mathrm{pllr},\mathrm{GFL},\mathrm{DFIG},7}\right)\,\left(\frac{99.502487562189\,\pi \,\Psi _{\mathrm{qr},\mathrm{GFL},\mathrm{DFIG},7}\,\mathrm{Sbase}\,f_{0}}{\mathrm{Lm}_{\mathrm{pu}}\,{\mathrm{Vbase}}^2}-\frac{100.497512437811\,\pi \,\Psi _{\mathrm{qs},\mathrm{GFL},\mathrm{DFIG},7}\,\mathrm{Sbase}\,f_{0}}{\mathrm{Lm}_{\mathrm{pu}}\,{\mathrm{Vbase}}^2}\right)-\sin\left(\theta _{\mathrm{pllr},\mathrm{GFL},\mathrm{DFIG},7}\right)\,\left(\frac{99.502487562189\,\pi \,\Psi _{\mathrm{dr},\mathrm{GFL},\mathrm{DFIG},7}\,\mathrm{Sbase}\,f_{0}}{\mathrm{Lm}_{\mathrm{pu}}\,{\mathrm{Vbase}}^2}-\frac{100.497512437811\,\pi \,\Psi _{\mathrm{ds},\mathrm{GFL},\mathrm{DFIG},7}\,\mathrm{Sbase}\,f_{0}}{\mathrm{Lm}_{\mathrm{pu}}\,{\mathrm{Vbase}}^2}\right)\right)}{\mathrm{Sbase}}-\frac{1.73205080756888\,\mathrm{Vbase}\,\left(i_{\mathrm{gq},\mathrm{GFL},\mathrm{DFIG},7}\,\cos\left(\theta _{\mathrm{pllg},\mathrm{GFL},\mathrm{DFIG},7}\right)-i_{\mathrm{gd},\mathrm{GFL},\mathrm{DFIG},7}\,\sin\left(\theta _{\mathrm{pllg},\mathrm{GFL},\mathrm{DFIG},7}\right)\right)}{\mathrm{Sbase}}\right)}{\mathrm{Vbase}}$
      | Automatically generated on 2025-11-01 18:34:17 .
  State_i_gd_GFL_DFIG_7_7f088 : Inport
  State_theta_pllg_GFL_DFIG_7_b67ea : Inport  Port=2
  State_i_gq_GFL_DFIG_7_cf5eb : Inport  Port=3
  State_theta_pllg_GFL_DFIG_7_36f0a : Inport  Port=4
  State_Psi_dr_GFL_DFIG_7_f818d : Inport  Port=5
  State_Psi_ds_GFL_DFIG_7_97cbe : Inport  Port=6
  State_theta_pllr_GFL_DFIG_7_9bdbf : Inport  Port=7
  State_Psi_qr_GFL_DFIG_7_bf209 : Inport  Port=8
  State_Psi_qs_GFL_DFIG_7_79723 : Inport  Port=9
  State_theta_pllr_GFL_DFIG_7_b0808 : Inport  Port=10
  Add_2e823 : Sum
  Add_4ecf3 : Sum
  Add_c306d : Sum
  Constant_-1_5a7ff : Constant  Value=-1
  Constant_-5.0_20d3f : Constant  Value=-5.0
  Constant_-99.502487562189_6e2de : Constant  Value=-99.502487562189
  Constant_-99.502487562189_b49f1 : Constant  Value=-99.502487562189
  Constant_1.73205080756888_27d7d : Constant  Value=1.73205080756888
  Constant_1.73205080756888_9e849 : Constant  Value=1.73205080756888
  Constant_10.0_0160e : Constant  Value=10.0
  Constant_100.497512437811_b319d : Constant  Value=100.497512437811
  Constant_100.497512437811_cc484 : Constant  Value=100.497512437811
  Constant_2.0_01f8a : Constant  Value=2.0
  Constant_2.0_2946a : Constant  Value=2.0
  Constant_2.0_58245 : Constant  Value=2.0
  Constant_2.0_c2e31 : Constant  Value=2.0
  Constant_3.45_4d8c8 : Constant  Value=3.45
  Constant_Lm_pu_1f8dd : Constant  Value=Lm_pu
  Constant_Lm_pu_2b48a : Constant  Value=Lm_pu
  Constant_Lm_pu_7b1a4 : Constant  Value=Lm_pu
  Constant_Lm_pu_a03f9 : Constant  Value=Lm_pu
  Constant_Sbase_03c53 : Constant  Value=Sbase
  Constant_Sbase_21ed6 : Constant  Value=Sbase
  Constant_Sbase_6366c : Constant  Value=Sbase
  Constant_Sbase_83789 : Constant  Value=Sbase
  Constant_Sbase_a7e3b : Constant  Value=Sbase
  Constant_Sbase_bc4aa : Constant  Value=Sbase
  Constant_Sbase_e2f93 : Constant  Value=Sbase
  Constant_Vbase_0ab6c : Constant  Value=Vbase
  Constant_Vbase_12217 : Constant  Value=Vbase
  Constant_Vbase_435cd : Constant  Value=Vbase
  Constant_Vbase_49856 : Constant  Value=Vbase
  Constant_Vbase_87f5c : Constant  Value=Vbase
  Constant_Vbase_a04ea : Constant  Value=Vbase
  Constant_Vbase_c199b : Constant  Value=Vbase
  Constant_f0_2845a : Constant  Value=f0
  Constant_f0_3f50d : Constant  Value=f0
  Constant_f0_60f2c : Constant  Value=f0
  Constant_f0_896c9 : Constant  Value=f0
  Constant_pi_6d0a9 : Constant  Value=pi
  Constant_pi_ac238 : Constant  Value=pi
  Constant_pi_da866 : Constant  Value=pi
  Constant_pi_e0915 : Constant  Value=pi
  Divide_0e81c : Product  Inputs=*/
  Divide_195cb : Product  Inputs=*/
  Divide_a1f0d : Product  Inputs=*/
  Divide_cac20 : Product  Inputs=*/
  Divide_d3556 : Product  Inputs=*/
  Divide_e0833 : Product  Inputs=*/
  Divide_f942a : Product  Inputs=*/
  MathFunc_cos_43560 : Trigonometry  Operator=cos
  MathFunc_cos_b477c : Trigonometry  Operator=cos
  MathFunc_sin_e7bc0 : Trigonometry
  MathFunc_sin_ea6d8 : Trigonometry
  Power_3033e : Math  Operator=pow
  Power_56a2e : Math  Operator=pow
  Power_8b7b1 : Math  Operator=pow
  Power_ab411 : Math  Operator=pow
  Power_ec6d9 : Math  Operator=pow
  Product_0b123 : Product
  Product_1eb50 : Product
  Product_22199 : Product
  Product_2f006 : Product
  Product_2fc93 : Product
  Product_32582 : Product
  Product_34eed : Product
  Product_3af3b : Product
  Product_3dea9 : Product
  Product_456ed : Product
  Product_4898a : Product
  Product_4b171 : Product
  Product_60092 : Product
  Product_65c37 : Product
  Product_6c2a0 : Product
  Product_6cc6d : Product
  Product_76e1b : Product
  Product_8a18d : Product
  Product_9792d : Product
  Product_9d0fa : Product
  Product_a8759 : Product
  Product_a92c5 : Product
  Product_b4ffc : Product
  Product_bb599 : Product
  Product_bd3dc : Product
  Product_c029a : Product
  Product_c092a : Product
  Product_c1071 : Product
  Product_c51eb : Product
  Product_c7a21 : Product
  Product_d573f : Product
  Product_f2961 : Product
  Subtract_2165d : Sum  Inputs=+-
  Subtract_9abf9 : Sum  Inputs=+-
  Blockout_i_q_GFL_DFIG_7_ec3de : Outport
  wires:
  Product_c029a/1 -> Product_9792d/1
  Constant_-99.502487562189_6e2de/1 -> Product_d573f/1
  Product_22199/1 -> Product_a8759/1
  Constant_100.497512437811_cc484/1 -> Product_c7a21/1
  Constant_pi_6d0a9/1 -> Product_d573f/2
  Divide_cac20/1 -> Add_c306d/1
  Constant_pi_e0915/1 -> Product_c7a21/2
  Constant_Sbase_6366c/1 -> Product_22199/2
  Constant_-99.502487562189_b49f1/1 -> Product_456ed/1
  Constant_100.497512437811_b319d/1 -> Product_f2961/1
  Constant_pi_ac238/1 -> Product_456ed/2
  Constant_pi_da866/1 -> Product_f2961/2
  Product_4898a/1 -> Product_60092/1
  Product_d573f/1 -> Product_bd3dc/1
  State_Psi_dr_GFL_DFIG_7_f818d/1 -> Product_bd3dc/2
  Product_c7a21/1 -> Product_6c2a0/1
  Product_9792d/1 -> Divide_cac20/1
  State_Psi_ds_GFL_DFIG_7_97cbe/1 -> Product_6c2a0/2
  Product_456ed/1 -> Product_8a18d/1
  State_Psi_qr_GFL_DFIG_7_bf209/1 -> Product_8a18d/2
  Product_f2961/1 -> Product_1eb50/1
  Product_3af3b/1 -> Divide_f942a/2
  State_Psi_qs_GFL_DFIG_7_79723/1 -> Product_1eb50/2
  Product_bd3dc/1 -> Product_9d0fa/1
  Constant_Lm_pu_7b1a4/1 -> Product_3dea9/1
  Constant_Sbase_83789/1 -> Product_9d0fa/2
  Product_2f006/1 -> Divide_cac20/2
  Constant_Vbase_435cd/1 -> Power_8b7b1/1
  Constant_Lm_pu_a03f9/1 -> Product_2f006/1
  Product_60092/1 -> Divide_e0833/1
  Constant_2.0_01f8a/1 -> Power_8b7b1/2
  Product_6c2a0/1 -> Product_65c37/1
  Constant_Sbase_bc4aa/1 -> Product_65c37/2
  Constant_Vbase_c199b/1 -> Power_3033e/1
  State_theta_pllg_GFL_DFIG_7_36f0a/1 -> MathFunc_cos_b477c/1
  Product_4b171/1 -> Divide_0e81c/2
  Constant_Lm_pu_1f8dd/1 -> Product_4b171/1
  Constant_2.0_58245/1 -> Power_3033e/2
  Product_8a18d/1 -> Product_c029a/1
  Power_ab411/1 -> Product_2fc93/2
  Constant_Sbase_21ed6/1 -> Product_c029a/2
  Divide_195cb/1 -> Add_4ecf3/2
  Constant_Vbase_87f5c/1 -> Power_ec6d9/1
  Constant_2.0_c2e31/1 -> Power_ec6d9/2
  Product_1eb50/1 -> Product_22199/1
  Constant_Vbase_12217/1 -> Power_56a2e/1
  State_theta_pllr_GFL_DFIG_7_9bdbf/1 -> MathFunc_sin_ea6d8/1
  Constant_2.0_2946a/1 -> Power_56a2e/2
  Product_9d0fa/1 -> Product_76e1b/1
  State_i_gd_GFL_DFIG_7_7f088/1 -> Product_c1071/2
  Constant_f0_896c9/1 -> Product_76e1b/2
  Constant_Lm_pu_2b48a/1 -> Product_3af3b/1
  Power_8b7b1/1 -> Product_3af3b/2
  Product_65c37/1 -> Product_c51eb/1
  Constant_f0_2845a/1 -> Product_c51eb/2
  Power_3033e/1 -> Product_3dea9/2
  Power_56a2e/1 -> Product_4b171/2
  Constant_f0_3f50d/1 -> Product_9792d/2
  Power_ec6d9/1 -> Product_2f006/2
  Constant_f0_60f2c/1 -> Product_a8759/2
  Product_76e1b/1 -> Divide_f942a/1
  Product_c51eb/1 -> Divide_195cb/1
  Product_3dea9/1 -> Divide_195cb/2
  Product_a8759/1 -> Divide_0e81c/1
  State_theta_pllg_GFL_DFIG_7_b67ea/1 -> MathFunc_sin_e7bc0/1
  Constant_-1_5a7ff/1 -> Product_c1071/1
  Divide_f942a/1 -> Add_4ecf3/1
  Divide_0e81c/1 -> Add_c306d/2
  State_theta_pllr_GFL_DFIG_7_b0808/1 -> MathFunc_cos_43560/1
  Product_c1071/1 -> Product_0b123/1
  MathFunc_sin_e7bc0/1 -> Product_0b123/2
  State_i_gq_GFL_DFIG_7_cf5eb/1 -> Product_bb599/1
  MathFunc_cos_b477c/1 -> Product_bb599/2
  Add_4ecf3/1 -> Product_6cc6d/1
  MathFunc_sin_ea6d8/1 -> Product_6cc6d/2
  Add_c306d/1 -> Product_b4ffc/1
  MathFunc_cos_43560/1 -> Product_b4ffc/2
  Constant_1.73205080756888_27d7d/1 -> Product_a92c5/1
  Constant_Vbase_0ab6c/1 -> Product_a92c5/2
  Product_0b123/1 -> Add_2e823/1
  Product_bb599/1 -> Add_2e823/2
  Constant_1.73205080756888_9e849/1 -> Product_c092a/1
  Subtract_2165d/1 -> Product_60092/2
  Constant_Vbase_49856/1 -> Product_c092a/2
  Product_6cc6d/1 -> Subtract_9abf9/1
  Product_b4ffc/1 -> Subtract_9abf9/2
  Constant_10.0_0160e/1 -> Power_ab411/1
  Constant_-5.0_20d3f/1 -> Power_ab411/2
  Product_a92c5/1 -> Product_34eed/1
  Add_2e823/1 -> Product_34eed/2
  Product_c092a/1 -> Product_32582/1
  Subtract_9abf9/1 -> Product_32582/2
  Constant_3.45_4d8c8/1 -> Product_2fc93/1
  Product_34eed/1 -> Divide_d3556/1
  Constant_Sbase_a7e3b/1 -> Divide_d3556/2
  Product_32582/1 -> Divide_a1f0d/1
  Constant_Sbase_e2f93/1 -> Divide_a1f0d/2
  Product_2fc93/1 -> Product_4898a/1
  Constant_Sbase_03c53/1 -> Product_4898a/2
  Divide_d3556/1 -> Subtract_2165d/1
  Divide_a1f0d/1 -> Subtract_2165d/2
  Constant_Vbase_a04ea/1 -> Divide_e0833/2
  Divide_e0833/1 -> Blockout_i_q_GFL_DFIG_7_ec3de/1

== system IEEE30_case/GFL_DFIG_7/w_r_GFL_DFIG_7_block ==
  note: w_r_GFL_DFIG_7 in IEEE30_case
      | $2\,\pi \,f_{0}-w_{m,\mathrm{GFL},\mathrm{DFIG},7}$
      | Automatically generated on 2025-11-01 18:34:29 .
  State_w_m_GFL_DFIG_7_cf772 : Inport
  Constant_2.0_345aa : Constant  Value=2.0
  Constant_f0_a71c3 : Constant  Value=f0
  Constant_pi_a880c : Constant  Value=pi
  Product_4a783 : Product
  Product_55ead : Product
  Subtract_7b422 : Sum  Inputs=+-
  Blockout_w_r_GFL_DFIG_7_71344 : Outport
  wires:
  Constant_2.0_345aa/1 -> Product_55ead/1
  Constant_f0_a71c3/1 -> Product_4a783/2
  Constant_pi_a880c/1 -> Product_55ead/2
  Product_55ead/1 -> Product_4a783/1
  State_w_m_GFL_DFIG_7_cf772/1 -> Subtract_7b422/2
  Product_4a783/1 -> Subtract_7b422/1
  Subtract_7b422/1 -> Blockout_w_r_GFL_DFIG_7_71344/1

== system IEEE30_case/SG_D_1/T_e_SG_D_1_block ==
  note: T_e_SG_D_1 in IEEE30_case
      | $-\frac{\psi _{d,\mathrm{SG},D,1}\,\left(\psi _{q,\mathrm{SG},D,1}+\frac{\psi _{\mathrm{gq},\mathrm{SG},D,1}\,\left(x_{l}-x_{\mathrm{qdd}}\right)}{x_{l}-x_{\mathrm{qd}}}+\frac{\psi _{\mathrm{kq},\mathrm{SG},D,1}\,\left(x_{\mathrm{qd}}-x_{\mathrm{qdd}}\right)}{x_{l}-x_{\mathrm{qd}}}\right)}{x_{\mathrm{qdd}}}-\frac{\psi _{q,\mathrm{SG},D,1}\,\left(\frac{\psi _{\mathrm{1d},\mathrm{SG},D,1}\,\left(x_{\mathrm{dd}}-x_{\mathrm{ddd}}\right)}{x_{\mathrm{dd}}-x_{l}}-\psi _{d,\mathrm{SG},D,1}+\frac{\psi _{\mathrm{fd},\mathrm{SG},D,1}\,\left(x_{\mathrm{ddd}}-x_{l}\right)}{x_{\mathrm{dd}}-x_{l}}\right)}{x_{\mathrm{ddd}}}$
      | Automatically generated on 2025-11-01 18:30:54 .
  State_psi_d_SG_D_1_f3ca8 : Inport
  State_psi_gq_SG_D_1_a6910 : Inport  Port=2
  State_psi_kq_SG_D_1_16b29 : Inport  Port=3
  State_psi_q_SG_D_1_15adc : Inport  Port=4
  State_psi_q_SG_D_1_53812 : Inport  Port=5
  State_psi_1d_SG_D_1_d6542 : Inport  Port=6
  State_psi_d_SG_D_1_e6af8 : Inport  Port=7
  State_psi_fd_SG_D_1_a9978 : Inport  Port=8
  Add_5e276 : Sum
  Add_75459 : Sum
  Add_b99d8 : Sum
  Add_c16c3 : Sum
  Add_cad1f : Sum
  Add_ffa83 : Sum
  Constant_-1_11454 : Constant  Value=-1
  Constant_-1_244dd : Constant  Value=-1
  Constant_-1_293a2 : Constant  Value=-1
  Constant_-1_314b4 : Constant  Value=-1
  Constant_-1_35d93 : Constant  Value=-1
  Constant_x_dd_3acd2 : Constant  Value=x_dd
  Constant_x_dd_6aa37 : Constant  Value=x_dd
  Constant_x_dd_de87e : Constant  Value=x_dd
  Constant_x_ddd_34f07 : Constant  Value=x_ddd
  Constant_x_ddd_7e6c2 : Constant  Value=x_ddd
  Constant_x_ddd_b57d1 : Constant  Value=x_ddd
  Constant_x_l_19b30 : Constant  Value=x_l
  Constant_x_l_1bea8 : Constant  Value=x_l
  Constant_x_l_61297 : Constant  Value=x_l
  Constant_x_l_a8e9a : Constant  Value=x_l
  Constant_x_l_be0ac : Constant  Value=x_l
  Constant_x_l_f30e0 : Constant  Value=x_l
  Constant_x_qd_5f156 : Constant  Value=x_qd
  Constant_x_qd_7db2c : Constant  Value=x_qd
  Constant_x_qd_cb987 : Constant  Value=x_qd
  Constant_x_qdd_1bc22 : Constant  Value=x_qdd
  Constant_x_qdd_3bc5e : Constant  Value=x_qdd
  Constant_x_qdd_edd7d : Constant  Value=x_qdd
  Divide_0a45e : Product  Inputs=*/
  Divide_61227 : Product  Inputs=*/
  Divide_de505 : Product  Inputs=*/
  Divide_eaf53 : Product  Inputs=*/
  Divide_efa34 : Product  Inputs=*/
  Divide_fbee8 : Product  Inputs=*/
  Product_219a4 : Product
  Product_6d92e : Product
  Product_842c2 : Product
  Product_876c4 : Product
  Product_9fabf : Product
  Product_a2506 : Product
  Product_a4b94 : Product
  Product_cf21b : Product
  Product_d9e39 : Product
  Product_e67cd : Product
  Product_ee13d : Product
  Subtract_15e20 : Sum  Inputs=+-
  Subtract_1c2a0 : Sum  Inputs=+-
  Subtract_7d77e : Sum  Inputs=+-
  Subtract_956be : Sum  Inputs=+-
  Subtract_95aa2 : Sum  Inputs=+-
  Subtract_ae172 : Sum  Inputs=+-
  Subtract_fde6f : Sum  Inputs=+-
  Blockout_T_e_SG_D_1_09252 : Outport
  wires:
  Product_ee13d/1 -> Divide_0a45e/1
  Product_9fabf/1 -> Add_ffa83/1
  Divide_0a45e/1 -> Subtract_95aa2/1
  Constant_-1_293a2/1 -> Product_9fabf/1
  Constant_x_l_a8e9a/1 -> Product_9fabf/2
  Constant_x_qdd_1bc22/1 -> Add_ffa83/2
  Constant_x_qd_5f156/1 -> Subtract_7d77e/1
  Constant_-1_314b4/1 -> Product_a4b94/1
  Constant_x_qdd_edd7d/1 -> Divide_efa34/2
  Constant_x_qdd_3bc5e/1 -> Subtract_7d77e/2
  State_psi_q_SG_D_1_53812/1 -> Product_e67cd/1
  Constant_x_dd_6aa37/1 -> Subtract_956be/1
  Constant_x_l_61297/1 -> Product_a4b94/2
  Subtract_956be/1 -> Product_842c2/2
  Constant_-1_11454/1 -> Product_cf21b/1
  Constant_x_l_1bea8/1 -> Product_cf21b/2
  Subtract_ae172/1 -> Product_e67cd/2
  State_psi_q_SG_D_1_15adc/1 -> Add_cad1f/2
  Constant_-1_35d93/1 -> Product_6d92e/1
  State_psi_1d_SG_D_1_d6542/1 -> Product_6d92e/2
  Constant_x_ddd_b57d1/1 -> Subtract_956be/2
  State_psi_gq_SG_D_1_a6910/1 -> Product_ee13d/1
  Add_ffa83/1 -> Product_ee13d/2
  Product_a4b94/1 -> Add_5e276/1
  Product_d9e39/1 -> Product_a2506/1
  Constant_x_qd_cb987/1 -> Add_5e276/2
  Product_842c2/1 -> Divide_de505/1
  State_psi_kq_SG_D_1_16b29/1 -> Product_876c4/1
  Add_5e276/1 -> Divide_0a45e/2
  Subtract_7d77e/1 -> Product_876c4/2
  Product_cf21b/1 -> Add_c16c3/1
  Constant_x_qd_7db2c/1 -> Add_c16c3/2
  Product_876c4/1 -> Divide_eaf53/1
  Product_6d92e/1 -> Product_842c2/1
  Constant_x_dd_de87e/1 -> Subtract_1c2a0/1
  Constant_x_l_be0ac/1 -> Subtract_1c2a0/2
  Constant_x_ddd_7e6c2/1 -> Subtract_fde6f/1
  Product_e67cd/1 -> Divide_fbee8/1
  Constant_x_l_19b30/1 -> Subtract_fde6f/2
  Divide_efa34/1 -> Add_b99d8/1
  Product_a2506/1 -> Divide_efa34/1
  Add_c16c3/1 -> Divide_eaf53/2
  Subtract_95aa2/1 -> Add_cad1f/1
  Divide_eaf53/1 -> Subtract_95aa2/2
  Subtract_1c2a0/1 -> Divide_de505/2
  State_psi_fd_SG_D_1_a9978/1 -> Product_219a4/1
  Constant_x_ddd_34f07/1 -> Divide_fbee8/2
  Subtract_fde6f/1 -> Product_219a4/2
  Constant_x_dd_3acd2/1 -> Subtract_15e20/1
  Constant_x_l_f30e0/1 -> Subtract_15e20/2
  Divide_de505/1 -> Add_75459/1
  Add_75459/1 -> Subtract_ae172/1
  State_psi_d_SG_D_1_e6af8/1 -> Add_75459/2
  Product_219a4/1 -> Divide_61227/1
  Subtract_15e20/1 -> Divide_61227/2
  Constant_-1_244dd/1 -> Product_d9e39/1
  State_psi_d_SG_D_1_f3ca8/1 -> Product_d9e39/2
  Divide_61227/1 -> Subtract_ae172/2
  Add_cad1f/1 -> Product_a2506/2
  Divide_fbee8/1 -> Add_b99d8/2
  Add_b99d8/1 -> Blockout_T_e_SG_D_1_09252/1

== system IEEE30_case/SG_D_1/d_E_fd_SG_D_1_block ==
  note: d_E_fd_SG_D_1 in IEEE30_case
      | $\frac{V_{f,\mathrm{SG},D,1}-E_{\mathrm{fd},\mathrm{SG},D,1}\,K_{E}}{T_{E}}$
      | Automatically generated on 2025-11-01 18:30:37 .
  State_E_fd_SG_D_1_d0430 : Inport
  State_V_f_SG_D_1_4243a : Inport  Port=2
  Add_a96d2 : Sum
  Constant_-1_551b1 : Constant  Value=-1
  Constant_K_E_82754 : Constant  Value=K_E
  Constant_T_E_2f014 : Constant  Value=T_E
  Divide_0edf1 : Product  Inputs=*/
  Product_41eb9 : Product
  Product_7c805 : Product
  Blockout_d_E_fd_SG_D_1_3912e : Outport
  wires:
  Add_a96d2/1 -> Divide_0edf1/1
  Constant_-1_551b1/1 -> Product_7c805/1
  State_E_fd_SG_D_1_d0430/1 -> Product_7c805/2
  Product_7c805/1 -> Product_41eb9/1
  Constant_K_E_82754/1 -> Product_41eb9/2
  Product_41eb9/1 -> Add_a96d2/1
  Constant_T_E_2f014/1 -> Divide_0edf1/2
  State_V_f_SG_D_1_4243a/1 -> Add_a96d2/2
  Divide_0edf1/1 -> Blockout_d_E_fd_SG_D_1_3912e/1

== system IEEE30_case/SG_D_1/d_Px_1_SG_D_1_block ==
  note: d_Px_1_SG_D_1 in IEEE30_case
      | $\frac{w_{\mathrm{SG},D,1}-2\,\pi \,f_{0}}{T_{w}}-\frac{\mathrm{Px}_{1,\mathrm{SG},D,1}}{T_{w}}$
      | Automatically generated on 2025-11-01 18:30:38 .
  State_Px_1_SG_D_1_b81ac : Inport
  State_w_SG_D_1_e905d : Inport  Port=2
  Add_7f51a : Sum
  Add_e904d : Sum
  Constant_-1_c83b3 : Constant  Value=-1
  Constant_-2.0_f594d : Constant  Value=-2.0
  Constant_T_w_11664 : Constant  Value=T_w
  Constant_T_w_e589a : Constant  Value=T_w
  Constant_f0_eaec2 : Constant  Value=f0
  Constant_pi_33d3b : Constant  Value=pi
  Divide_05e15 : Product  Inputs=*/
  Divide_6b24c : Product  Inputs=*/
  Product_324f0 : Product
  Product_b2a0b : Product
  Product_e8bed : Product
  Blockout_d_Px_1_SG_D_1_1380a : Outport
  wires:
  Add_7f51a/1 -> Blockout_d_Px_1_SG_D_1_1380a/1
  Constant_-2.0_f594d/1 -> Product_b2a0b/1
  Product_324f0/1 -> Divide_05e15/1
  State_w_SG_D_1_e905d/1 -> Add_e904d/2
  Constant_-1_c83b3/1 -> Product_324f0/1
  Constant_f0_eaec2/1 -> Product_e8bed/2
  Constant_pi_33d3b/1 -> Product_b2a0b/2
  Product_e8bed/1 -> Add_e904d/1
  Product_b2a0b/1 -> Product_e8bed/1
  State_Px_1_SG_D_1_b81ac/1 -> Product_324f0/2
  Constant_T_w_e589a/1 -> Divide_05e15/2
  Add_e904d/1 -> Divide_6b24c/1
  Constant_T_w_11664/1 -> Divide_6b24c/2
  Divide_05e15/1 -> Add_7f51a/1
  Divide_6b24c/1 -> Add_7f51a/2
